simulink model "ltc2422_task"  (Simulink 3.00)
libraries: mathlib x4, arclib x2, speclib x1

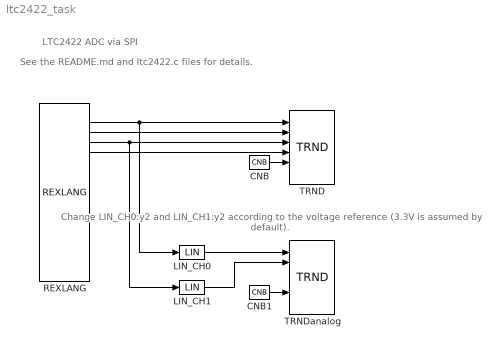
== system ltc2422_task ==
  note: Change LIN_CH0:y2 and LIN_CH1:y2 according
      | to the voltage reference (3.3V is assumed by default).
  note: See the README.md and ltc2422.c files for details.
  note: LTC2422 ADC via SPI
  CNB : mathlib/CNB  YCN=on
  CNB1 : mathlib/CNB  YCN=on
  LIN_CH0 : mathlib/LIN  u1=0  y1=0  u2=1048575  y2=3.3
  LIN_CH1 : mathlib/LIN  u1=0  y1=0  u2=1048575  y2=3.3
  REXLANG : speclib/REXLANG  strs=0  SystemSampleTime=-1  tab_matlab=BASIC  srcname=ltc2422.c  srctype=1: C-like  stack=0  debug=1: No check  p0=/dev/spidev0.0  p1=0  p2=0  p3=0  p4=0  p5=0  p6=0  p7=0  p8=0  p9=0  p10=0  p11=0  p12=0  p13=0  p14=0  p15=0  fname=/dev/spidev0.0
  TRND : arclib/TRND  n=4  l=1000  btype=8: Double  ptype1=1: Store  ptype2=1: Store  ptype3=1: Store  ptype4=1: Store  pfac=1  afac=0  arc=0  id=1  Title=ADC data  timesrc=1
  TRNDanalog : arclib/TRND  n=4  l=1000  btype=8: Double  ptype1=1: Store  ptype2=1: Store  ptype3=1: Store  ptype4=1: Store  pfac=1  afac=0  arc=0  id=2  Title=Analog values  timesrc=1
  wires:
  CNB/1 -> TRND/5
  CNB1/1 -> TRNDanalog/5
  LIN_CH0/1 -> TRNDanalog/1
  LIN_CH1/1 -> TRNDanalog/2
  REXLANG/2 -> LIN_CH0/1, TRND/1
  REXLANG/3 -> TRND/2
  REXLANG/4 -> LIN_CH1/1, TRND/3
  REXLANG/5 -> TRND/4
